simulink model "tran_mdl_demo_v14"  (Simulink 7.0)
settings: Solver=ode3  StartTime=0.0  StopTime=100  FixedStep=0.001  RelTol=1e-3
PreLoadFcn:
  | eng_mdl_demo_v14_setup
InitFcn:
  | eng_mdl_demo_v14_setup
undefined symbols (not defined in the file or in its folder): notex
libraries: hil14_mdl_lib x1, ni_annotations_lib x1
CloseFcn:
  | eng_mdl_demo_v14_close
settings Model: Creator=Eric Bradley  LastModifiedBy=blueuser
settings OptimizationCC: SimCompilerOptimization=On
settings DebuggingCC: InheritedTsInSrcMsg=none  ParameterPrecisionLossMsg=none
settings RTWCC: SystemTargetFile=NIVeriStand.tlc  TemplateMakefile=NIVeriStand_vc.tmf  Description=NI VeriStand Real-Time Target for Release 2007b or later  ProcessScript=NIVeriStand_make_rtw_hook
settings STFCustomTargetCC: GenFloatMathFcnCalls=ANSI_C  MatFileLogging=on  SystemTargetFile=NIVeriStand.tlc
settings CustomProperty: Value=on
settings EnumStrPairs: String=Default

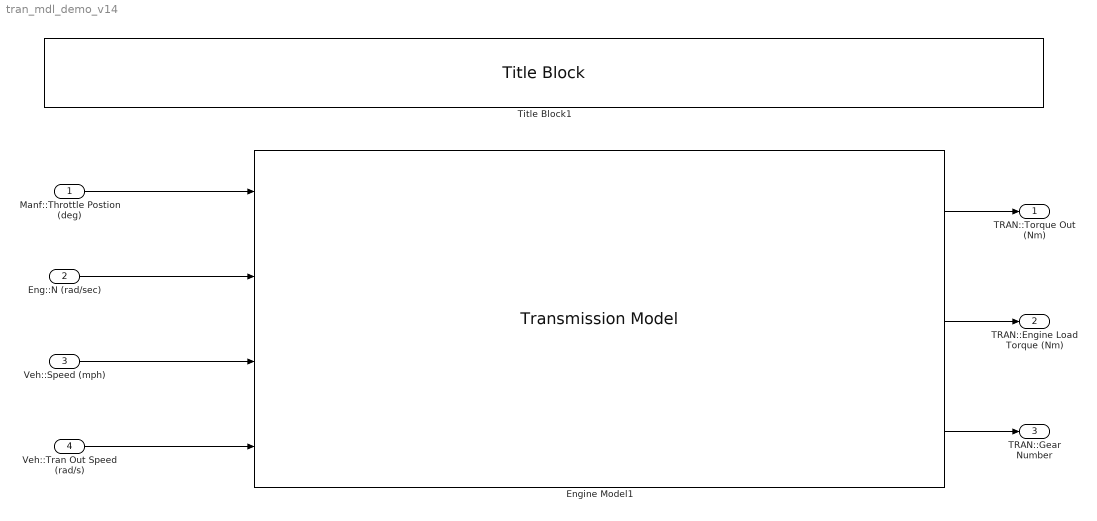
== system tran_mdl_demo_v14 ==
  Manf::Throttle Postion (deg) : Inport  OutDataType=sfix(16)  OutScaling=2^0
  Eng::N (rad/sec) : Inport  Port=2  OutDataType=sfix(16)  OutScaling=2^0
  Veh::Speed (mph) : Inport  Port=3  OutDataType=sfix(16)  OutScaling=2^0
  Veh::Tran Out Speed (rad/s) : Inport  Port=4  OutDataType=sfix(16)  OutScaling=2^0
  Engine Model1 : hil14_mdl_lib/Transmission Model  SystemSampleTime=-1  iname='tran.jpg'  scale=0.375
  Title Block1 : ni_annotations_lib/Title Block  SystemSampleTime=-1  tx_title=notex(get_param(gcs,'Name'))
  TRAN::Torque Out (Nm) : Outport  OutDataType=sfix(16)  OutScaling=2^0
  TRAN::Engine Load Torque (Nm) : Outport  Port=2  OutDataType=sfix(16)  OutScaling=2^0
  TRAN::Gear Number : Outport  Port=3  OutDataType=sfix(16)  OutScaling=2^0
  wires:
  Manf::Throttle Postion (deg)/1 -> Engine Model1/1
  Eng::N (rad/sec)/1 -> Engine Model1/2
  Veh::Speed (mph)/1 -> Engine Model1/3
  Veh::Tran Out Speed (rad/s)/1 -> Engine Model1/4
  Engine Model1/1 -> TRAN::Torque Out (Nm)/1
  Engine Model1/2 -> TRAN::Engine Load Torque (Nm)/1
  Engine Model1/3 -> TRAN::Gear Number/1
